simulink subsystem "FTC_UnknownV2"  (R2022a)
settings: Solver=VariableStepAuto  StartTime=0.0  StopTime=10.0  RelTol=1e-3
values from neighbouring files (symbols this model uses):
  g = (9.8)    (= 9.8)    [H250_LOEKnown_400HzParam.m]    (also in H250_LOEUnknown_400HzParam.m; H333_LOEKnown_400HzParam.m)
  J = (diag([0.0056 0.0056 0.0104]))    [H250_LOEKnown_400HzParam.m]    (also in H250_LOEUnknown_400HzParam.m; H333_LOEKnown_400HzParam.m = (diag([0.012 0.0120 0.02])))
  M = ([ 1          1          1         1 ... (first row only)    [H250_LOEKnown_400HzParam.m]    (also in H250_LOEUnknown_400HzParam.m; H333_LOEKnown_400HzParam.m)
  m = (0.752)    (= 0.752)    [H250_LOEKnown_400HzParam.m]    (also in H250_LOEUnknown_400HzParam.m; H333_LOEKnown_400HzParam.m = 1.13)
  MY_ATT_P = Pixhawk_CSC.Parameter( {single(8), 'MY_ATT_P'}  )    [H250_LOEKnown_400HzParam.m]    (also in H250_LOEUnknown_400HzParam.m = Pixhawk_CSC.Parameter( {single(3), 'MY_ATT_P'}  ); H333_LOEKnown_400HzParam.m)
  MY_ATT_P_YAW = Pixhawk_CSC.Parameter( {single(0), 'MY_ATT_P_YAW'}  )    [H250_LOEKnown_400HzParam.m]    (also in H250_LOEUnknown_400HzParam.m = Pixhawk_CSC.Parameter( {single(0.0), 'MY_ATT_P_YAW'}  ); H333_LOEKnown_400HzParam.m)
  MY_K_CP = Pixhawk_CSC.Parameter({single(0.7), 'MY_K_CP'} )    [H250_LOEUnknown_400HzParam.m]
  MY_POS_P = Pixhawk_CSC.Parameter( {single(0.5), 'MY_POS_P'}  )    [H250_LOEKnown_400HzParam.m]    (also in H250_LOEUnknown_400HzParam.m; H333_LOEKnown_400HzParam.m)
  MY_RATE_P = Pixhawk_CSC.Parameter( {single(12), 'MY_RATE_P'}  )    [H250_LOEKnown_400HzParam.m]    (also in H250_LOEUnknown_400HzParam.m = Pixhawk_CSC.Parameter( {single(14), 'MY_RATE_P'}  ); H333_LOEKnown_400HzParam.m)
  MY_RATE_P_YAW = Pixhawk_CSC.Parameter( {single(0.3), 'MY_RATE_P_YAW'}  )    [H250_LOEKnown_400HzParam.m]    (also in H250_LOEUnknown_400HzParam.m = Pixhawk_CSC.Parameter( {single(0.0), 'MY_RATE_P_YAW'}  ); H333_LOEKnown_400HzParam.m)
  MY_SAT_AD = Pixhawk_CSC.Parameter({single(0.13), 'MY_SAT_AD'} )    [H250_LOEKnown_400HzParam.m]    (also in H250_LOEUnknown_400HzParam.m; H333_LOEKnown_400HzParam.m)
  MY_TAU_P_A = Pixhawk_CSC.Parameter( {single(0), 'MY_TAU_P_A'}  )    [H250_LOEKnown_400HzParam.m]    (also in H250_LOEUnknown_400HzParam.m = Pixhawk_CSC.Parameter( {single(0.0), 'MY_TAU_P_A'}  ); H333_LOEKnown_400HzParam.m)
  MY_TAU_P_A_YAW = Pixhawk_CSC.Parameter( {single(0), 'MY_TAU_P_A_YAW'}  )    [H250_LOEKnown_400HzParam.m]    (also in H250_LOEUnknown_400HzParam.m; H333_LOEKnown_400HzParam.m)
  MY_TAU_P_P = Pixhawk_CSC.Parameter( {single(1.5), 'MY_TAU_P_P'}  )    [H250_LOEKnown_400HzParam.m]    (also in H250_LOEUnknown_400HzParam.m = Pixhawk_CSC.Parameter( {single(1.3), 'MY_TAU_P_P'}  ); H333_LOEKnown_400HzParam.m)
  MY_TAU_P_P_YAW = Pixhawk_CSC.Parameter( {single(0.1), 'MY_TAU_P_P_YAW'}  )    [H250_LOEKnown_400HzParam.m]    (also in H250_LOEUnknown_400HzParam.m; H333_LOEKnown_400HzParam.m)
  MY_VEL_P = Pixhawk_CSC.Parameter( {single(0.8), 'MY_VEL_P'}  )    [H250_LOEKnown_400HzParam.m]    (also in H250_LOEUnknown_400HzParam.m; H333_LOEKnown_400HzParam.m)
  T00 = single([m*g/4 m*g/4 m*g/4 m*g/4]')    [H250_LOEKnown_400HzParam.m]    (also in H250_LOEUnknown_400HzParam.m; H333_LOEKnown_400HzParam.m)
  Tf = 0.06    [H250_LOEKnown_400HzParam.m]    (also in H250_LOEUnknown_400HzParam.m; H333_LOEKnown_400HzParam.m)
  Tmotorbar = (0.035)    (= 0.035)    [H250_LOEKnown_400HzParam.m]    (also in H250_LOEUnknown_400HzParam.m = 0.032; H333_LOEKnown_400HzParam.m)
  Ts = 1/400    (= 0.0025)    [H250_LOEKnown_400HzParam.m]    (also in H250_LOEUnknown_400HzParam.m; H333_LOEKnown_400HzParam.m)
undefined symbols (not defined in the file or in its folder): MY_POS_ALT, MY_VEL_ALT
libraries: discretizing x14, slpidlib x4, simulink x2, pixhawk_slib_uORB_RW x1
settings Model: Creator=kcx06  LastModifiedBy=kcx06
settings SolverCC: AlgebraicLoopSolver=TrustRegion
settings DebuggingCC: UnconnectedInputMsg=warning  UnconnectedOutputMsg=warning  UnconnectedLineMsg=warning  SFMachineParentedDataDiag=warning
settings RTWCC: DLArmComputeVersion=19.05

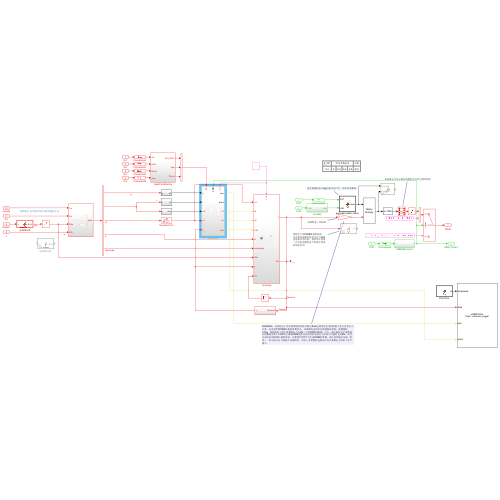
[thumbnail: Simulink's stored preview of the top-level diagram]
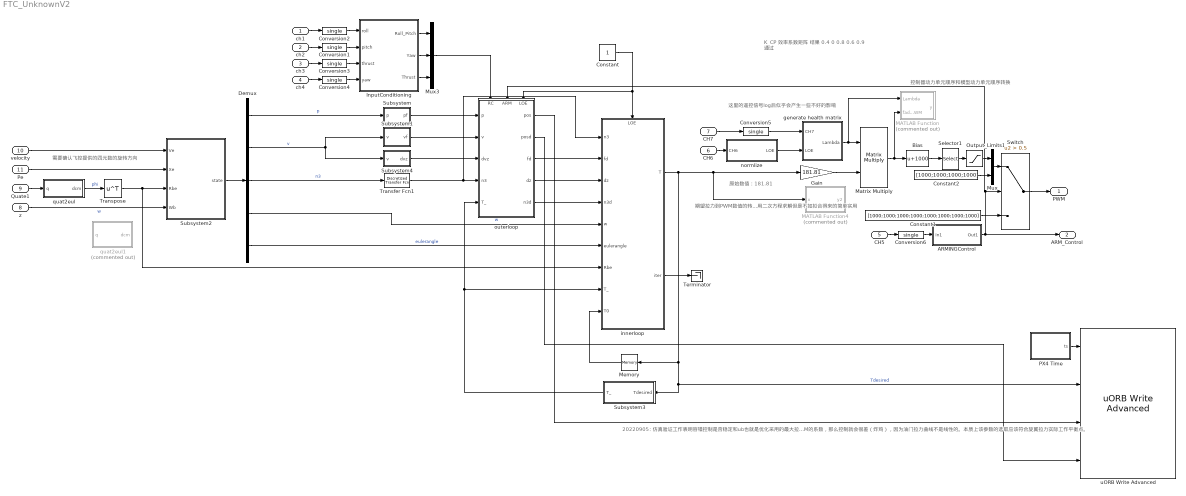
== system FTC_UnknownV2 ==
  note: 这里的遥控信号log后似乎会产生一些不好的影响
  note: K_CP
      | 效率系数矩阵
      | 结果
      |
      | 0.4
      | 0
      | 0.8
      | 0.6
      | 0.9
      | 通过
  note: 20220905：仿真验证工作表明容错控制是否稳定和ub也就是优化采用的最大拉力没有太大关系。而是和T到PWM转换的系数有关，该系数的选取更可能遵循该原则：旋翼整机0.7kg，故障情况下每个旋翼的拉力为2N（大约PWM=1400）左右，那么乘以这个系数的后的数值再加上1000所生成的PWM值所对应的实际电机拉力应该尽可能的也是2N。所以在实际采用8.5N上限的时候，如果使用117作为生成PWM的系数，那么控制就会很差（炸鸡），因为油门拉力曲线不是线性的。本质上该参数的选取应该符合旋翼拉力实际工作平衡点。
  note: 期望拉力到PWM数值的转换，该关系是根据电机油门拉力数据直接拟合得出的。虽然可以使用二次方程求解但是不如拟合得来的简单实用
  note: 原始数值：181.81
  note: 需要确认飞控提供的四元数的旋转方向
  note: 控制器动力单元顺序和模型动力单元顺序转换
  ch1 : Inport  OutDataTypeStr=uint16  PortDimensions=1
  ch2 : Inport  Port=2  OutDataTypeStr=uint16  PortDimensions=1
  ch3 : Inport  Port=3  OutDataTypeStr=uint16  PortDimensions=1
  ch4 : Inport  Port=4  OutDataTypeStr=uint16  PortDimensions=1
  CH5 : Inport  Port=5  OutDataTypeStr=uint16  PortDimensions=1  Interpolate=off
  CH6 : Inport  Port=6
  CH7 : Inport  Port=7
  z : Inport  Port=8
  Quate1 : Inport  Port=9
  velocity : Inport  Port=10
  Pe : Inport  Port=11
  ARMINGControl : Subsystem
  Bias : Bias  Bias=1000  SaturateOnIntegerOverflow=off
  Constant : Constant  OutDataTypeStr=single
  Constant1 : Constant  Value=[1000;1000;1000;1000;1000;1000;1000;1000]  OutDataTypeStr=single
  Constant2 : Constant  Value=[1000;1000;1000;1000]  OutDataTypeStr=single
  Conversion{1..6} (6 alike) : DataTypeConversion  OutDataTypeStr=single  SaturateOnIntegerOverflow=off  RndMeth=Floor
  Demux : Demux  Outputs=[3 3 3 3 3]
  Gain : Gain  Gain=181.81  OutDataTypeStr=single
  InputConditioning : Subsystem
  MATLAB Function : MATLAB Function  Commented=on  TreatAsAtomicUnit=on
  MATLAB Function4 : MATLAB Function  Commented=on  TreatAsAtomicUnit=on
  Matrix Multiply : Product  Multiplication=Matrix(*)
  Memory : Memory  InitialCondition=T00
  Mux : Mux  Inputs=2
  Mux3 : Mux  Inputs=3
  Output_Limits1 : Saturate  UpperLimit=2000  LowerLimit=1000
  PX4 Time : MATLAB Function  TreatAsAtomicUnit=on
  Selector1 : Selector  IndexMode=Zero-based  InputPortWidth=4  IndexOptions=Index vector (dialog)  Indices=[0 2 3 1]  OutputSizes=1
  Subsystem : Subsystem
  Subsystem1 : Subsystem
  Subsystem2 : Subsystem
  Subsystem3 : Subsystem
  Subsystem4 : Subsystem
  Switch : Switch  Criteria=u2 > Threshold  Threshold=0.5  SaturateOnIntegerOverflow=off  InputSameDT=off
  Terminator : Terminator
  Transfer Fcn1 : discretizing/Discretized Transfer Fcn  Numerator=[1]  Denominator=[Tf 1]  AbsTol=auto  SampleTime=Ts  method=zoh  Wc=1
      link override Discrete Transfer Fcn: InitialStates=[0;0;1]
      settings: SourceProductBaseCode=SL
  Transpose : Math  Operator=transpose
  generate health matrix : MATLAB Function  TreatAsAtomicUnit=on
  innerloop : Subsystem
      settings: PortSchema="{\"entries\":[{\"content\":{\"sides\":[{\"content\":{\"connectorIds\":[\"In1\",\"In2\",\"In3\",\"In4\",\"In5\",\"In6\",\"In7\",\"In8\",\"In9\"]},\"type\":\"ConnectorPlacement.EquallySpacedRectSide\",\"uuid\":\"43c6e1bd-c98b-47b4-98da-f51fdffff433\"},{\"content\":{\"connectorIds\":[\"Out1\",\"Out2\"],\"side\":\"RIGHT\"},\"type\":\"ConnectorPlacement.EquallySpacedRectSide\",\"uuid\":\"ac1c9532-9168-4bf4-8fed-08d3fdc16453\"},{\"content\":{\"connectorIds\":[\"In10\"],\"side\":\"TOP\"},\"type\":\"ConnectorPlacement.EquallySpacedRectSide\",\"uuid\":\"32774b13-030c-47c6-b846-fc6c0ce2dd6f\"}]},\"type\":\"ConnectorPlacement.EquallySpacedConnector\",\"uuid\":\"dd62421a-d766-429a-a161-5a0f77c5a7ba\"}],\"packageUris\":[\"http://schema.mathworks.com/mf0/Connector/R2020b\"],\"version\":\"1.0\"}"
  normlize : Subsystem
  outerloop : Subsystem
      settings: PortSchema="{\"entries\":[{\"content\":{\"sides\":[{\"content\":{\"connectorIds\":[\"In1\",\"In2\",\"In3\",\"In4\",\"In5\"]},\"type\":\"ConnectorPlacement.EquallySpacedRectSide\",\"uuid\":\"59983f3e-2daf-41bd-bc3f-074c85f4b2eb\"},{\"content\":{\"connectorIds\":[\"Out1\",\"Out2\",\"Out3\",\"Out4\",\"Out5\"],\"side\":\"RIGHT\"},\"type\":\"ConnectorPlacement.EquallySpacedRectSide\",\"uuid\":\"6ee11e40-7870-4737-b9e6-fd7c25119100\"},{\"content\":{\"connectorIds\":[\"In6\",\"In7\",\"In8\"],\"side\":\"TOP\"},\"type\":\"ConnectorPlacement.EquallySpacedRectSide\",\"uuid\":\"847e9a02-4621-4cf8-a675-1479afa28be0\"}]},\"type\":\"ConnectorPlacement.EquallySpacedConnector\",\"uuid\":\"28981c41-e87e-4da3-ac2d-04a56d75ff2b\"}],\"packageUris\":[\"http://schema.mathworks.com/mf0/Connector/R2020b\"],\"version\":\"1.0\"}"
  quat2eul : MATLAB Function  TreatAsAtomicUnit=on
  quat2eul1 : MATLAB Function  Commented=on  TreatAsAtomicUnit=on
  uORB Write Advanced : pixhawk_slib_uORB_RW/uORB Write Advanced  Ts=0  uORB_AdvtQueue=on  uORB_FieldEnabledArr="0  0  0  1  0  0  0  0  0  0  0"  uORB_Topic_str=0  uORB_Struct_DT="[1  1  1  1  1]"  BlockInputCount=5  uORB_StructParams="[\"voltage_v\",\"voltage_filtered_v\",\"current_a\",\"current_filtered_a\",\"remaining\"]"  uORB_PortSizes="[1  1  1  1]"  MsgSizeOf=0  MW_update=true
      settings: SourceProductName=Pixhawk Target Blocks
  PWM : Outport  PortDimensions=8  VectorParamsAs1DForOutWhenUnconnected=off
  ARM_Control : Outport  Port=2  PortDimensions=1  VectorParamsAs1DForOutWhenUnconnected=off
  wires:
  CH6/1 -> normlize/1(CH6)
  InputConditioning/3(Thrust) -> Mux3/3
  velocity/1 -> Subsystem2/1(Ve)
  Conversion2/1 -> InputConditioning/1(roll)
  Transpose/1 -> innerloop/7(Rbe), Subsystem2/3(Rbe)
  Demux/3 -> Transfer Fcn1/1  "n3"
  InputConditioning/1(Roll_Pitch) -> Mux3/1
  outerloop/4(dz) -> innerloop/3(dz)
  Constant/1 -> outerloop/8(LOE), innerloop/10(LOE)
  Constant1/1 -> Switch/3
  Subsystem3/1(T_) -> outerloop/5(T_), innerloop/8(T_)
  quat2eul/1(dcm) -> Transpose/1  "phi"
  z/1 -> Subsystem2/4(Wb)  "w"
  Conversion3/1 -> InputConditioning/3(thrust)
  Pe/1 -> Subsystem2/2(Xe)
  CH5/1 -> Conversion6/1
  Quate1/1 -> quat2eul/1(q)
  Demux/2 -> Subsystem1/1(v), Subsystem4/1(v)  "v"
  ch4/1 -> Conversion4/1
  Output_Limits1/1 -> Mux/1
  Demux/4 -> innerloop/5(w)  "w"
  outerloop/3(fd) -> innerloop/2(fd)
  Memory/1 -> innerloop/9(T0)
  Demux/5 -> innerloop/6(eulerangle)  "eulerangle"
  ch1/1 -> Conversion2/1
  InputConditioning/2(Yaw) -> Mux3/2
  Selector1/1 -> Output_Limits1/1
  innerloop/1(T) -> Subsystem3/1(Tdesired), uORB Write Advanced/2, Memory/1, Gain/1, MATLAB Function4/1(x)  "Tdesired"
  ch2/1 -> Conversion1/1
  Conversion4/1 -> InputConditioning/4(yaw)
  normlize/1(LOE) -> generate health matrix/2(LOE)
  Mux/1 -> Switch/1
  Subsystem2/1(state) -> Demux/1
  Conversion6/1 -> ARMINGControl/1(In1)
  Switch/1 -> PWM/1
  ch3/1 -> Conversion3/1
  ARMINGControl/1(Out1) -> outerloop/7(ARM), Switch/2, ARM_Control/1
  Mux3/1 -> outerloop/6(RC)
  Constant2/1 -> Mux/2
  Conversion1/1 -> InputConditioning/2(pitch)
  outerloop/5(n3d) -> innerloop/4(n3d)
  Demux/1 -> Subsystem/1(p)  "p"
  Subsystem/1(pf) -> outerloop/1(p)
  Subsystem1/1(vf) -> outerloop/2(v)
  Subsystem4/1(dvz) -> outerloop/3(dvz)
  Transfer Fcn1/1 -> innerloop/1(n3), outerloop/4(n3)
  PX4 Time/1(ts) -> uORB Write Advanced/1
  innerloop/2(iter) -> Terminator/1
  outerloop/1(pos) -> uORB Write Advanced/3
  outerloop/2(posd) -> uORB Write Advanced/4
  Matrix Multiply/1 -> MATLAB Function/2(fadePWM), Bias/1
  Gain/1 -> Matrix Multiply/2
  generate health matrix/1(Lambda) -> MATLAB Function/1(Lambda), Matrix Multiply/1
  CH7/1 -> Conversion5/1
  Conversion5/1 -> generate health matrix/1(CH7)
  Bias/1 -> Selector1/1

== system FTC_UnknownV2/ARMINGControl ==
  In1 : Inport
  Compare To Constant3 : simulink/Logic and Bit Operations/Compare To Constant  relop=>=  const=uint16(1500)  OutDataTypeStr=boolean
  Out1 : Outport  VectorParamsAs1DForOutWhenUnconnected=off
  wires:
  In1/1 -> Compare To Constant3/1
  Compare To Constant3/1 -> Out1/1

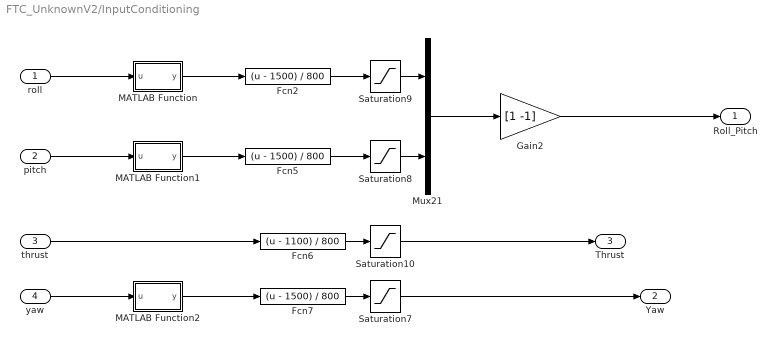
== system FTC_UnknownV2/InputConditioning ==
  roll : Inport
  pitch : Inport  Port=2
  thrust : Inport  Port=3
  yaw : Inport  Port=4
  Fcn2 : Fcn  Expr=(u - 1500) / 800
  Fcn5 : Fcn  Expr=(u - 1500) / 800
  Fcn6 : Fcn  Expr=(u - 1100) / 800
  Fcn7 : Fcn  Expr=(u - 1500) / 800
  Gain2 : Gain  Gain=[1 -1]  OutDataTypeStr=Inherit: Inherit via back propagation
  MATLAB Function : MATLAB Function  TreatAsAtomicUnit=on
  MATLAB Function1 : MATLAB Function  TreatAsAtomicUnit=on
  MATLAB Function2 : MATLAB Function  TreatAsAtomicUnit=on
  Mux21 : Mux  Inputs=2
  Saturation10 : Saturate  UpperLimit=1  LowerLimit=0
  Saturation7 : Saturate  UpperLimit=1  LowerLimit=-1
  Saturation8 : Saturate  UpperLimit=1  LowerLimit=-1
  Saturation9 : Saturate  UpperLimit=1  LowerLimit=-1
  Roll_Pitch : Outport  VectorParamsAs1DForOutWhenUnconnected=off
  Yaw : Outport  Port=2  VectorParamsAs1DForOutWhenUnconnected=off
  Thrust : Outport  Port=3  VectorParamsAs1DForOutWhenUnconnected=off
  wires:
  yaw/1 -> MATLAB Function2/1(u)
  MATLAB Function/1(y) -> Fcn2/1
  MATLAB Function1/1(y) -> Fcn5/1
  roll/1 -> MATLAB Function/1(u)
  thrust/1 -> Fcn6/1
  MATLAB Function2/1(y) -> Fcn7/1
  pitch/1 -> MATLAB Function1/1(u)
  Fcn7/1 -> Saturation7/1
  Saturation9/1 -> Mux21/1
  Fcn5/1 -> Saturation8/1
  Fcn2/1 -> Saturation9/1
  Fcn6/1 -> Saturation10/1
  Saturation8/1 -> Mux21/2
  Mux21/1 -> Gain2/1
  Gain2/1 -> Roll_Pitch/1
  Saturation7/1 -> Yaw/1
  Saturation10/1 -> Thrust/1

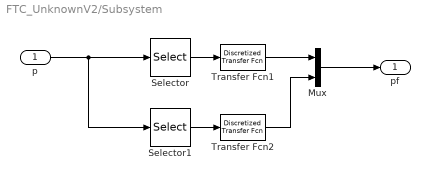
== system FTC_UnknownV2/Subsystem ==
  p : Inport
  Mux : Mux  Inputs=2
  Selector : Selector  IndexMode=Zero-based  InputPortWidth=3  IndexOptions=Index vector (dialog)  Indices=[0 1]  OutputSizes=1
  Selector1 : Selector  IndexMode=Zero-based  InputPortWidth=3  IndexOptions=Index vector (dialog)  Indices=[2]  OutputSizes=1
  Transfer Fcn1 : discretizing/Discretized Transfer Fcn  Numerator=[1 ]  Denominator=[Tf 1]  AbsTol=auto  SampleTime=Ts  method=zoh  Wc=1
      settings: SourceProductBaseCode=SL
  Transfer Fcn2 : discretizing/Discretized Transfer Fcn  Numerator=[1 ]  Denominator=[Tf 1]  AbsTol=auto  SampleTime=Ts  method=zoh  Wc=1
      settings: SourceProductBaseCode=SL
  pf : Outport
  wires:
  Transfer Fcn1/1 -> Mux/1
  Selector/1 -> Transfer Fcn1/1
  Transfer Fcn2/1 -> Mux/2
  Selector1/1 -> Transfer Fcn2/1
  Mux/1 -> pf/1
  p/1 -> Selector/1, Selector1/1

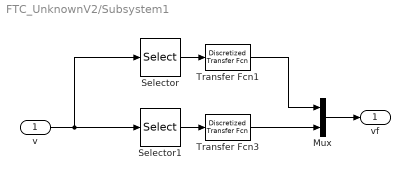
== system FTC_UnknownV2/Subsystem1 ==
  v : Inport
  Mux : Mux  Inputs=2
  Selector : Selector  IndexMode=Zero-based  InputPortWidth=3  IndexOptions=Index vector (dialog)  Indices=[0 1]  OutputSizes=1
  Selector1 : Selector  IndexMode=Zero-based  InputPortWidth=3  IndexOptions=Index vector (dialog)  Indices=[2]  OutputSizes=1
  Transfer Fcn1 : discretizing/Discretized Transfer Fcn  Numerator=[1 ]  Denominator=[Tf 1]  AbsTol=auto  SampleTime=Ts  method=zoh  Wc=1
      settings: SourceProductBaseCode=SL
  Transfer Fcn3 : discretizing/Discretized Transfer Fcn  Numerator=[1 ]  Denominator=[Tf 1]  AbsTol=auto  SampleTime=Ts  method=zoh  Wc=1
      settings: SourceProductBaseCode=SL
  vf : Outport
  wires:
  Transfer Fcn1/1 -> Mux/1
  Selector/1 -> Transfer Fcn1/1
  Mux/1 -> vf/1
  v/1 -> Selector1/1, Selector/1
  Selector1/1 -> Transfer Fcn3/1
  Transfer Fcn3/1 -> Mux/2

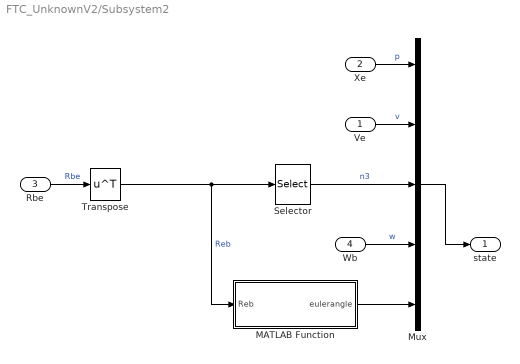
== system FTC_UnknownV2/Subsystem2 ==
  Ve : Inport
  Xe : Inport  Port=2
  Rbe : Inport  Port=3
  Wb : Inport  Port=4
  MATLAB Function : MATLAB Function  TreatAsAtomicUnit=on
  Mux : Mux  Inputs=[3 3 3 3 3]
  Selector : Selector  NumberOfDimensions=2  IndexMode=Zero-based  InputPortWidth=3  IndexOptions=Select all,Index vector (dialog)  Indices=[1 3],2  OutputSizes=1,1
  Transpose : Math  Operator=transpose
  state : Outport
  wires:
  Transpose/1 -> MATLAB Function/1(Reb), Selector/1  "Reb"
  Xe/1 -> Mux/1  "p"
  Ve/1 -> Mux/2  "v"
  Wb/1 -> Mux/4  "w"
  Selector/1 -> Mux/3  "n3"
  Rbe/1 -> Transpose/1  "Rbe"
  MATLAB Function/1(eulerangle) -> Mux/5
  Mux/1 -> state/1

== system FTC_UnknownV2/Subsystem3 ==
  Tdesired : Inport
  Transfer Fcn10 : discretizing/Discretized Transfer Fcn  Numerator=[1]  Denominator=[Tmotorbar 1]  AbsTol=auto  SampleTime=Ts  method=zoh  Wc=1
      settings: SourceProductBaseCode=SL
  Transfer Fcn9 : discretizing/Discretized Transfer Fcn  Numerator=[1]  Denominator=[Tf 1]  AbsTol=auto  SampleTime=Ts  method=zoh  Wc=1
      settings: SourceProductBaseCode=SL
  T_ : Outport
  wires:
  Transfer Fcn9/1 -> Transfer Fcn10/1
  Tdesired/1 -> Transfer Fcn9/1
  Transfer Fcn10/1 -> T_/1

== system FTC_UnknownV2/Subsystem4 ==
  v : Inport
  Selector2 : Selector  IndexMode=Zero-based  InputPortWidth=3  IndexOptions=Index vector (dialog)  Indices=[2]  OutputSizes=1
  Transfer Fcn : discretizing/Discretized Transfer Fcn  Numerator=[1 0]  Denominator=[Tf 1]  AbsTol=auto  SampleTime=Ts  method=zoh  Wc=1
      settings: SourceProductBaseCode=SL
  dvz : Outport
  wires:
  Transfer Fcn/1 -> dvz/1
  v/1 -> Selector2/1
  Selector2/1 -> Transfer Fcn/1

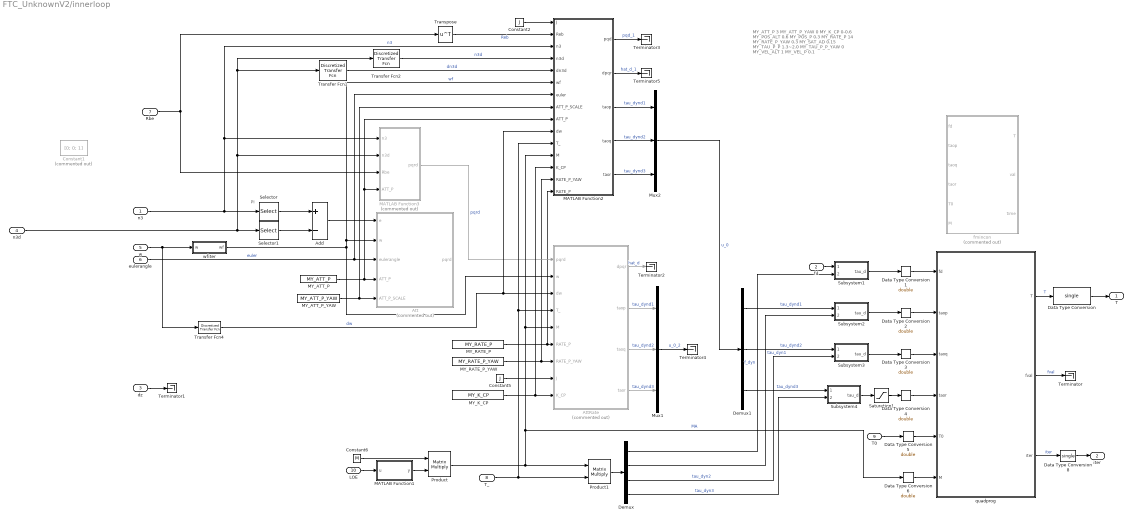
== system FTC_UnknownV2/innerloop ==
  note: PI
  note: MY_ATT_P
      | 3
      |
      | MY_ATT_P_YAW
      | 0
      |
      | MY_K_CP
      | 0-0.6
      |
      | MY_POS_ALT
      | 0.6
      |
      | MY_POS_P
      | 0.3
      |
      | MY_RATE_P
      | 14
      |
      | MY_RATE_P_YAW
      | 0.3
      |
      | MY_SAT_AD
      | 0.15
      |
      | MY_TAU_P_P
      | 1.3~2.0
      |
      | MY_TAU_P_P_YAW
      | 0
      |
      | MY_VEL_ALT
      | 1
      |
      | MY_VEL_P
      | 0.1
  n3 : Inport
  fd : Inport  Port=2
  dz : Inport  Port=3
  n3d : Inport  Port=4
  w : Inport  Port=5
  eulerangle : Inport  Port=6
  Rbe : Inport  Port=7
  T_ : Inport  Port=8
  T0 : Inport  Port=9
  LOE : Inport  Port=10
  Add : Sum  Inputs=+-
  Att : MATLAB Function  Commented=on  TreatAsAtomicUnit=on
  AttRate : MATLAB Function  Commented=on  TreatAsAtomicUnit=on
  Constant1 : Constant  Commented=on  Value=[0; 0; 1]
  Constant2 : Constant  Value=J  OutDataTypeStr=single
  Constant5 : Constant  Value=J  OutDataTypeStr=single
  Constant6 : Constant  Value=M  OutDataTypeStr=single
  Data Type Conversion : DataTypeConversion  OutDataTypeStr=single  SaturateOnIntegerOverflow=off  RndMeth=Floor
  Data Type Conversion{1..6} (6 alike) : DataTypeConversion  OutDataTypeStr=double  SaturateOnIntegerOverflow=off  RndMeth=Floor
  Data Type Conversion8 : DataTypeConversion  OutDataTypeStr=single  SaturateOnIntegerOverflow=off  RndMeth=Floor
  Demux : Demux
  Demux1 : Demux  Outputs=3
  MATLAB Function1 : MATLAB Function  TreatAsAtomicUnit=on
  MATLAB Function2 : MATLAB Function  TreatAsAtomicUnit=on
  MATLAB Function3 : MATLAB Function  Commented=on  TreatAsAtomicUnit=on
  MY_ATT_P : Constant  Value=MY_ATT_P
  MY_ATT_P_YAW : Constant  Value=MY_ATT_P_YAW
  MY_K_CP : Constant  Value=MY_K_CP
  MY_RATE_P : Constant  Value=MY_RATE_P
  MY_RATE_P_YAW : Constant  Value=MY_RATE_P_YAW
  Mux1 : Mux  Inputs=3
  Mux2 : Mux  Inputs=3
  Product : Product  Multiplication=Matrix(*)
  Product1 : Product  Multiplication=Matrix(*)
  Saturation1 : Saturate  UpperLimit=0.075  LowerLimit=-0.075
  Selector : Selector  IndexMode=Zero-based  InputPortWidth=3  IndexOptions=Index vector (dialog)  Indices=[0 1]  OutputSizes=1
  Selector1 : Selector  IndexMode=Zero-based  InputPortWidth=3  IndexOptions=Index vector (dialog)  Indices=[0 1]  OutputSizes=1
  Subsystem1 : Subsystem
  Subsystem2 : Subsystem
  Subsystem3 : Subsystem
  Subsystem4 : Subsystem
  Terminator{,1..5} (6 alike) : Terminator
  Transfer Fcn1 : discretizing/Discretized Transfer Fcn  Numerator=[1 0]  Denominator=[Tf 1]  AbsTol=auto  SampleTime=Ts  method=zoh  Wc=1
      settings: SourceProductBaseCode=SL
  Transfer Fcn2 : discretizing/Discretized Transfer Fcn  Numerator=[1]  Denominator=[Tf 1]  AbsTol=auto  SampleTime=Ts  method=zoh  Wc=1
      link override Discrete Transfer Fcn: InitialStates=[0;0;1]
      settings: SourceProductBaseCode=SL
  Transfer Fcn4 : discretizing/Discretized Transfer Fcn  Numerator=[1 0]  Denominator=[Tf 1]  AbsTol=auto  SampleTime=Ts  method=zoh  Wc=1
      settings: SourceProductBaseCode=SL
  Transpose : Math  Operator=transpose
  fmincon : MATLAB Function  Commented=on  TreatAsAtomicUnit=on
  quadprog : MATLAB Function  TreatAsAtomicUnit=on
  wfiter : Subsystem
  T : Outport  PortDimensions=4
  iter : Outport  Port=2
  wires:
  Mux1/1 -> Terminator4/1  "u_0_2"
  MATLAB Function2/1(pqd) -> Terminator3/1  "pqd_1"
  AttRate/1(dpqr) -> Terminator2/1  "hat_d"
  Mux2/1 -> Demux1/1  "u_0"
  MATLAB Function2/5(taor) -> Mux2/3  "tau_dynd3"
  MATLAB Function2/4(taoq) -> Mux2/2  "tau_dynd2"
  MATLAB Function2/3(taop) -> Mux2/1  "tau_dynd1"
  AttRate/2(taop) -> Mux1/1  "tau_dynd1"
  AttRate/3(taoq) -> Mux1/2  "tau_dynd2"
  AttRate/4(taor) -> Mux1/3  "tau_dynd3"
  Constant2/1 -> MATLAB Function2/1(J)
  Transpose/1 -> MATLAB Function2/2(Reb)  "Reb"
  dz/1 -> Terminator1/1
  Selector/1 -> Add/1
  Selector1/1 -> Add/2
  Rbe/1 -> MATLAB Function3/3(Rbe), Transpose/1
  n3d/1 -> Selector1/1, MATLAB Function3/2(n3d), Transfer Fcn2/1, Transfer Fcn1/1
  MY_ATT_P_YAW/1 -> Att/5(ATT_P_SCALE), MATLAB Function2/8(ATT_P_SCALE)
  MY_ATT_P/1 -> Att/4(ATT_P), MATLAB Function2/9(ATT_P), MATLAB Function3/4(ATT_P)
  MY_RATE_P_YAW/1 -> AttRate/7(RATE_P_YAW), MATLAB Function2/14(RATE_P_YAW)
  MY_RATE_P/1 -> AttRate/6(RATE_P), MATLAB Function2/15(RATE_P)
  Data Type Conversion/1 -> T/1
  MATLAB Function1/1(y) -> Product/2
  MATLAB Function3/1(pqrd) -> AttRate/1(pqrd)  "pqrd"
  Product1/1 -> Demux/1
  n3/1 -> MATLAB Function2/3(n3), MATLAB Function3/1(n3), Selector/1  "n3"
  Product/1 -> Product1/1, AttRate/5(M), MATLAB Function2/12(M), Data Type Conversion6/1  "MA"
  LOE/1 -> MATLAB Function1/1(u)
  Demux/4 -> Subsystem4/2(tau_dyn)  "tau_dyn3"
  Demux1/3 -> Subsystem4/1(tau_dynd)  "tau_dynd3"
  Demux/3 -> Subsystem3/2(tau_dyn)  "tau_dyn2"
  Demux1/2 -> Subsystem3/1(tau_dynd)  "tau_dynd2"
  Demux/2 -> Subsystem2/2(tau_dyn)  "tau_dyn1"
  Demux1/1 -> Subsystem2/1(tau_dynd)  "tau_dynd1"
  fd/1 -> Subsystem1/1(tau_dynd)
  Demux/1 -> Subsystem1/2(tau_dyn)  "f_dyn"
  Data Type Conversion8/1 -> iter/1
  quadprog/3(iter) -> Data Type Conversion8/1  "iter"
  Subsystem4/1(tau_d) -> Saturation1/1
  Data Type Conversion6/1 -> quadprog/6(M)
  Data Type Conversion5/1 -> quadprog/5(T0)
  Data Type Conversion4/1 -> quadprog/4(taor)
  Data Type Conversion3/1 -> quadprog/3(taoq)
  Data Type Conversion2/1 -> quadprog/2(taop)
  Data Type Conversion1/1 -> quadprog/1(fd)
  quadprog/1(T) -> Data Type Conversion/1  "T"
  wfiter/1(wf) -> AttRate/2(w), Att/2(w), MATLAB Function2/6(wf)  "wf"
  w/1 -> Transfer Fcn4/1, wfiter/1(w)
  eulerangle/1 -> Att/3(eulerangle), MATLAB Function2/7(euler)  "euler"
  quadprog/2(fval) -> Terminator/1  "fval"
  Constant6/1 -> Product/1
  Constant5/1 -> AttRate/8(J)
  T_/1 -> AttRate/4(T_), MATLAB Function2/11(T_), Product1/2
  T0/1 -> Data Type Conversion5/1
  MATLAB Function2/2(dpqr) -> Terminator5/1  "hat_d_1"
  Transfer Fcn4/1 -> AttRate/3(dw), MATLAB Function2/10(dw)  "dw"
  MY_K_CP/1 -> AttRate/9(K_CP), MATLAB Function2/13(K_CP)
  Add/1 -> Att/1(e)
  Subsystem1/1(tau_d) -> Data Type Conversion1/1
  Subsystem2/1(tau_d) -> Data Type Conversion2/1
  Subsystem3/1(tau_d) -> Data Type Conversion3/1
  Saturation1/1 -> Data Type Conversion4/1
  Transfer Fcn2/1 -> MATLAB Function2/4(n3d)  "n3d"
  Transfer Fcn1/1 -> MATLAB Function2/5(dn3d)  "dn3d"

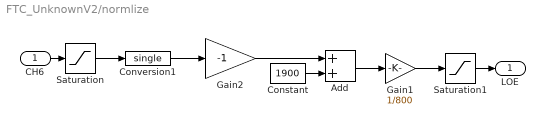
== system FTC_UnknownV2/normlize ==
  CH6 : Inport
  Add : Sum
  Constant : Constant  Value=1900  OutDataTypeStr=single
  Conversion1 : DataTypeConversion  OutDataTypeStr=single  SaturateOnIntegerOverflow=off  RndMeth=Floor
  Gain1 : Gain  Gain=1/800
  Gain2 : Gain  Gain=-1
  Saturation : Saturate  UpperLimit=1900  LowerLimit=1100
  Saturation1 : Saturate  UpperLimit=1  LowerLimit=0
  LOE : Outport
  wires:
  Saturation1/1 -> LOE/1
  Conversion1/1 -> Gain2/1
  Constant/1 -> Add/2
  CH6/1 -> Saturation/1
  Add/1 -> Gain1/1
  Gain1/1 -> Saturation1/1
  Gain2/1 -> Add/1
  Saturation/1 -> Conversion1/1

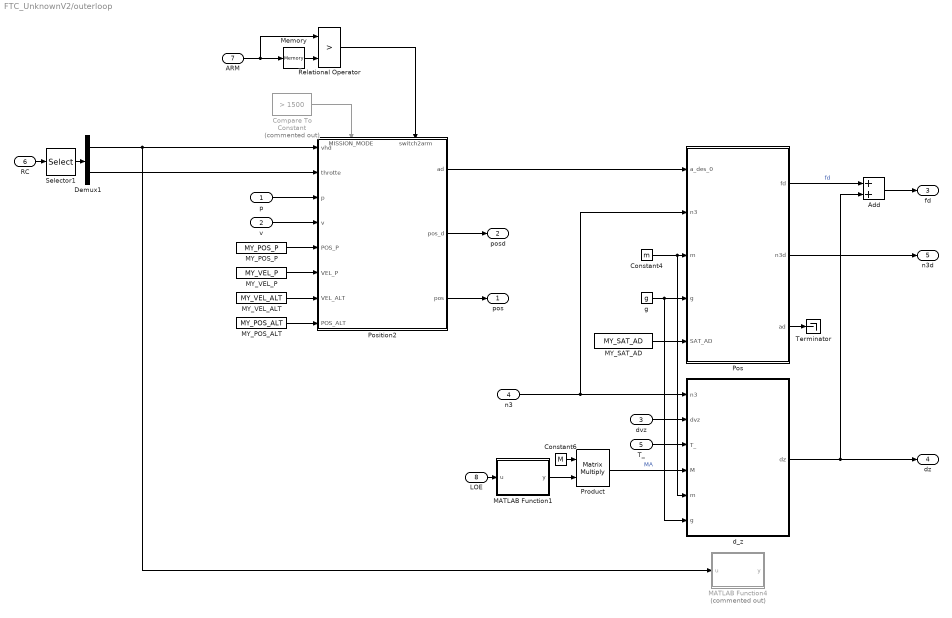
== system FTC_UnknownV2/outerloop ==
  p : Inport
  v : Inport  Port=2
  dvz : Inport  Port=3
  n3 : Inport  Port=4
  T_ : Inport  Port=5
  RC : Inport  Port=6
  ARM : Inport  Port=7
  LOE : Inport  Port=8
  Add : Sum
  Compare To Constant : simulink/Logic and Bit Operations/Compare To Constant  Commented=on  relop=>  const=1500  OutDataTypeStr=boolean
  Constant4 : Constant  Value=m  OutDataTypeStr=single
  Constant6 : Constant  Value=M  OutDataTypeStr=single
  Demux1 : Demux  Outputs=[2 1]
  MATLAB Function1 : MATLAB Function  TreatAsAtomicUnit=on
  MATLAB Function4 : MATLAB Function  Commented=on  TreatAsAtomicUnit=on
  MY_POS_ALT : Constant  Value=MY_POS_ALT
  MY_POS_P : Constant  Value=MY_POS_P
  MY_SAT_AD : Constant  Value=MY_SAT_AD
      settings: AttributesFormatString=|
      | 0.13
      | Default
  MY_VEL_ALT : Constant  Value=MY_VEL_ALT
  MY_VEL_P : Constant  Value=MY_VEL_P
  Memory : Memory  InheritSampleTime=on
  Pos : MATLAB Function  TreatAsAtomicUnit=on
  Position2 : Subsystem
      settings: PortSchema="{\"entries\":[{\"content\":{\"sides\":[{\"content\":{\"connectorIds\":[\"In1\",\"In2\",\"In3\",\"In4\",\"In5\",\"In6\",\"In7\",\"In8\"]},\"type\":\"ConnectorPlacement.EquallySpacedRectSide\",\"uuid\":\"60776ec6-01a0-44f3-b730-3d7732f047d0\"},{\"content\":{\"connectorIds\":[\"Out1\",\"Out2\",\"Out3\"],\"side\":\"RIGHT\"},\"type\":\"ConnectorPlacement.EquallySpacedRectSide\",\"uuid\":\"42b0027c-881e-456b-a4a1-739d1f8a7516\"},{\"content\":{\"connectorIds\":[\"In9\",\"In10\"],\"side\":\"TOP\"},\"type\":\"ConnectorPlacement.EquallySpacedRectSide\",\"uuid\":\"cc212ab2-5a31-41d0-b525-290641d80c94\"}]},\"type\":\"ConnectorPlacement.EquallySpacedConnector\",\"uuid\":\"907853b4-a5dd-49ed-90eb-6ed189df5e2d\"}],\"packageUris\":[\"http://schema.mathworks.com/mf0/Connector/R2020b\"],\"version\":\"1.0\"}"
  Product : Product  Multiplication=Matrix(*)
  Relational Operator : RelationalOperator  Operator=>  OutDataTypeStr=boolean  RndMeth=Simplest  InputSameDT=off
  Selector1 : Selector  IndexMode=Zero-based  InputPortWidth=4  IndexOptions=Index vector (dialog)  Indices=[1 0 3]  OutputSizes=1
  Terminator : Terminator
  d_z : MATLAB Function  TreatAsAtomicUnit=on
  g : Constant  Value=g  OutDataTypeStr=single
  pos : Outport
  posd : Outport  Port=2
  fd : Outport  Port=3
  dz : Outport  Port=4
  n3d : Outport  Port=5
  wires:
  Pos/2(n3d) -> n3d/1
  Relational Operator/1 -> Position2/10(switch2arm)
  Memory/1 -> Relational Operator/2
  ARM/1 -> Memory/1, Relational Operator/1
  Compare To Constant/1 -> Position2/9(MISSION_MODE)
  MY_POS_ALT/1 -> Position2/8(POS_ALT)
  MY_VEL_ALT/1 -> Position2/7(VEL_ALT)
  dvz/1 -> d_z/2(dvz)
  p/1 -> Position2/3(p)
  v/1 -> Position2/4(v)
  MY_SAT_AD/1 -> Pos/5(SAT_AD)
  MY_VEL_P/1 -> Position2/6(VEL_P)
  MY_POS_P/1 -> Position2/5(POS_P)
  Demux1/1 -> MATLAB Function4/1(u), Position2/1(vhd)
  Position2/1(ad) -> Pos/1(a_des_0)
  RC/1 -> Selector1/1
  Product/1 -> d_z/4(M)  "MA"
  Constant6/1 -> Product/1
  LOE/1 -> MATLAB Function1/1(u)
  MATLAB Function1/1(y) -> Product/2
  n3/1 -> d_z/1(n3), Pos/2(n3)
  d_z/1(dz) -> Add/2, dz/1
  Add/1 -> fd/1
  g/1 -> d_z/6(g), Pos/4(g)
  Constant4/1 -> d_z/5(m), Pos/3(m)
  T_/1 -> d_z/3(T_)
  Pos/1(fd) -> Add/1  "fd"
  Position2/2(pos_d) -> posd/1
  Position2/3(pos) -> pos/1
  Pos/3(ad) -> Terminator/1
  Selector1/1 -> Demux1/1
  Demux1/2 -> Position2/2(throtte)

== system FTC_UnknownV2/innerloop/Subsystem1 ==
  tau_dynd : Inport
  tau_dyn : Inport  Port=2
  Gain7 : Gain
  Sum1 : Sum  Inputs=|++
  Sum4 : Sum  Inputs=|+-
  tau_d : Outport
  wires:
  tau_dyn/1 -> Sum4/2, Sum1/2
  Sum1/1 -> tau_d/1
  Sum4/1 -> Gain7/1
  Gain7/1 -> Sum1/1
  tau_dynd/1 -> Sum4/1  "omega"

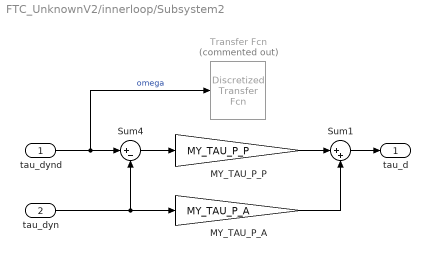
== system FTC_UnknownV2/innerloop/Subsystem2 ==
  tau_dynd : Inport
  tau_dyn : Inport  Port=2
  MY_TAU_P_A : Gain  Gain=MY_TAU_P_A
  MY_TAU_P_P : Gain  Gain=MY_TAU_P_P
  Sum1 : Sum  Inputs=|++
  Sum4 : Sum  Inputs=|+-
  Transfer Fcn : discretizing/Discretized Transfer Fcn  Commented=on  Numerator=[0.005 0]  Denominator=[Tf 1]  AbsTol=auto  SampleTime=Ts  method=zoh  Wc=1
      settings: SourceProductBaseCode=SL
  tau_d : Outport
  wires:
  MY_TAU_P_P/1 -> Sum1/1
  MY_TAU_P_A/1 -> Sum1/2
  tau_dynd/1 -> Sum4/1, Transfer Fcn/1  "omega"
  Sum4/1 -> MY_TAU_P_P/1
  Sum1/1 -> tau_d/1
  tau_dyn/1 -> MY_TAU_P_A/1, Sum4/2

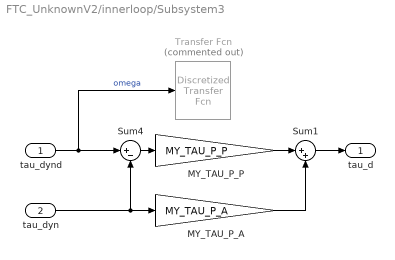
== system FTC_UnknownV2/innerloop/Subsystem3 ==
  tau_dynd : Inport
  tau_dyn : Inport  Port=2
  MY_TAU_P_A : Gain  Gain=MY_TAU_P_A
  MY_TAU_P_P : Gain  Gain=MY_TAU_P_P
  Sum1 : Sum  Inputs=|++
  Sum4 : Sum  Inputs=|+-
  Transfer Fcn : discretizing/Discretized Transfer Fcn  Commented=on  Numerator=[0.005 0]  Denominator=[Tf 1]  AbsTol=auto  SampleTime=Ts  method=zoh  Wc=1
      settings: SourceProductBaseCode=SL
  tau_d : Outport
  wires:
  MY_TAU_P_P/1 -> Sum1/1
  MY_TAU_P_A/1 -> Sum1/2
  tau_dyn/1 -> MY_TAU_P_A/1, Sum4/2
  Sum1/1 -> tau_d/1
  Sum4/1 -> MY_TAU_P_P/1
  tau_dynd/1 -> Sum4/1, Transfer Fcn/1  "omega"

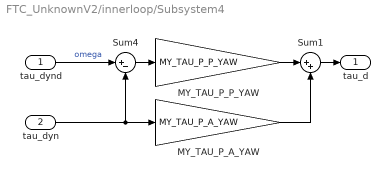
== system FTC_UnknownV2/innerloop/Subsystem4 ==
  tau_dynd : Inport
  tau_dyn : Inport  Port=2
  MY_TAU_P_A_YAW : Gain  Gain=MY_TAU_P_A_YAW
  MY_TAU_P_P_YAW : Gain  Gain=MY_TAU_P_P_YAW
  Sum1 : Sum  Inputs=|++
  Sum4 : Sum  Inputs=|+-
  tau_d : Outport
  wires:
  MY_TAU_P_A_YAW/1 -> Sum1/2
  tau_dynd/1 -> Sum4/1  "omega"
  MY_TAU_P_P_YAW/1 -> Sum1/1
  Sum4/1 -> MY_TAU_P_P_YAW/1
  Sum1/1 -> tau_d/1
  tau_dyn/1 -> Sum4/2, MY_TAU_P_A_YAW/1

== system FTC_UnknownV2/innerloop/wfiter ==
  w : Inport
  Transfer Fcn4 : discretizing/Discretized Transfer Fcn  Numerator=[1]  Denominator=[Tf 1]  AbsTol=auto  SampleTime=Ts  method=zoh  Wc=1
      settings: SourceProductBaseCode=SL
  wf : Outport
  wires:
  w/1 -> Transfer Fcn4/1
  Transfer Fcn4/1 -> wf/1

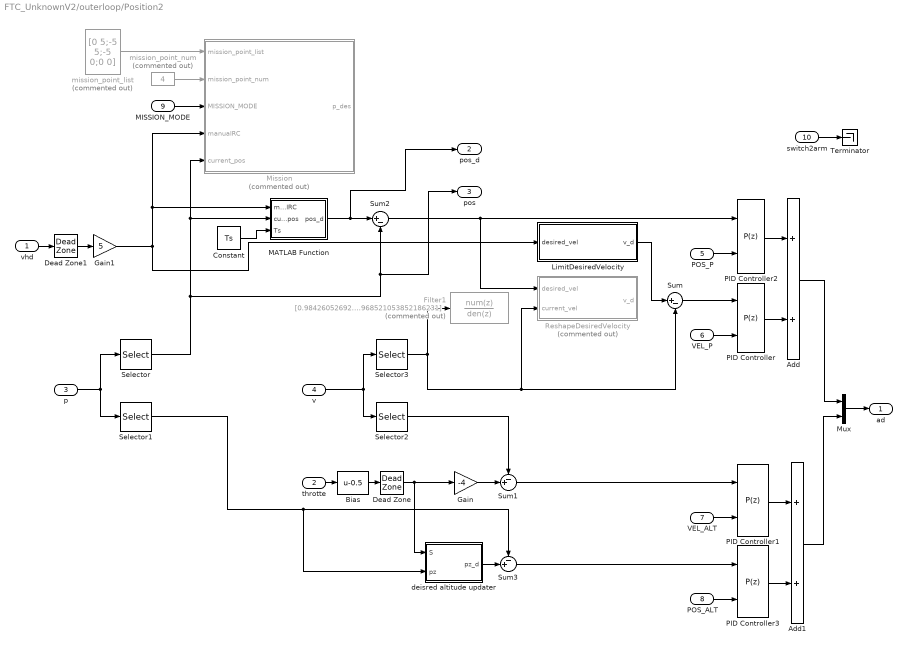
== system FTC_UnknownV2/outerloop/Position2 ==
  vhd : Inport
  throtte : Inport  Port=2
  p : Inport  Port=3
  v : Inport  Port=4
  POS_P : Inport  Port=5
  VEL_P : Inport  Port=6
  VEL_ALT : Inport  Port=7
  POS_ALT : Inport  Port=8
  MISSION_MODE : Inport  Port=9
  switch2arm : Inport  Port=10
  Add : Sum
  Add1 : Sum
  Bias : Bias  Bias=-0.5  SaturateOnIntegerOverflow=off
  Constant : Constant  Value=Ts  OutDataTypeStr=single
  Dead Zone : DeadZone  LowerValue=-0.1  UpperValue=0.1
  Dead Zone1 : DeadZone  LowerValue=-0.1  UpperValue=0.1
  Filter1 : DiscreteFilter  Tag=BlockMethodSubSystem  Commented=on  Numerator=[0.984260526926093116 -1.90667634508841477 0.984260526926093116]  Denominator=[1 -1.90667634508841477 0.968521053852186231]  SampleTime=1/100  a0EqualsOne=on
  Gain : Gain  Gain=-4
  Gain1 : Gain  Gain=5
  LimitDesiredVelocity : MATLAB Function  TreatAsAtomicUnit=on
  MATLAB Function : MATLAB Function  TreatAsAtomicUnit=on
  Mission : Stateflow chart  Commented=on  TreatAsAtomicUnit=on
  Mux : Mux  Inputs=2
  PID Controller{,1..3} (4 alike) : slpidlib/PID Controller  Controller=P  Form=Parallel  TimeDomain=Discrete-time  UseExternalTs=off  SampleTime=-1  IntegratorMethod=Forward Euler  FilterMethod=Forward Euler  ControllerParametersSource=external  P=1  I=1  UseKiTs=on  D=0  N=100  UseFilter=on  TunerSelectOption=Transfer Function Based (PID Tuner App)  InitialConditionSource=internal  InitialConditionForIntegrator=0  InitialConditionForFilter=0  DifferentiatorICPrevScaledInput=0  ExternalReset=none  TrackingMode=off  Kt=1  LimitOutput=off  SatLimitsSource=internal  UpperSaturationLimit=1  LowerSaturationLimit=-1  LinearizeAsGain=on  AntiWindupMode=clamping  Kb=1  POutMin=[]  POutMax=[]  IOutMin=[]  IOutMax=[]  DOutMin=[]  DOutMax=[]  NOutMin=[]  NOutMax=[]  SumOutMin=[]  SumOutMax=[]  SaturationOutMin=[]  SaturationOutMax=[]  PParamMin=[]  PParamMax=[]  IParamMin=[]  IParamMax=[]  DParamMin=[]  DParamMax=[]  NParamMin=[]  NParamMax=[]  KbParamMin=[]  KbParamMax=[]  KtParamMin=[]  KtParamMax=[]  KbOutMin=[]  KbOutMax=[]  KtOutMin=[]  KtOutMax=[]  IntegratorOutMin=[]  IntegratorOutMax=[]  FilterOutMin=[]  FilterOutMax=[]  SumI1OutMin=[]  SumI1OutMax=[]  SumI2OutMin=[]  SumI2OutMax=[]  SumI3OutMin=[]  SumI3OutMax=[]  SumI4OutMin=[]  SumI4OutMax=[]  SumDOutMin=[]  SumDOutMax=[]  DifferentiatorOutMin=[]  DifferentiatorOutMax=[]  FilterDiffOutCoefMin=[]  FilterDiffOutCoefMax=[]  ReciprocalOutMin=[]  ReciprocalOutMax=[]  SumDenOutMin=[]  SumDenOutMax=[]  SumNumOutMin=[]  SumNumOutMax=[]  DivideOutMin=[]  DivideOutMax=[]  UdiffTsProdOutMin=[]  UdiffTsProdOutMax=[]  NTsProdOutMin=[]  NTsProdOutMax=[]  UintegralTsProdOutMin=[]  UintegralTsProdOutMax=[]  UngainTsProdOutMin=[]  UngainTsProdOutMax=[]  IntegratorContinuousStateAttributes=''  IntegratorStateMustResolveToSignalObject=off  IntegratorRTWStateStorageClass=Auto  FilterContinuousStateAttributes=''  FilterStateMustResolveToSignalObject=off  FilterRTWStateStorageClass=Auto  ParallelPVariant=ExternalParameters  IdealPVariant=Disabled  IVariant=Disabled  DVariant=Disabled  IntegratorVariant=Disabled  SatVariant=Disabled  AWVariant=Disabled  PCopyVariant=Disabled  TRVariant=Disabled  FdbkBlocksVariant=Forward  IdealPFdbkVariant=Disabled  SatFdbkVariant=Disabled  DerivativeFilterVariant=Disabled  NVariant=Disabled  NCopyVariant=Disabled_SignalSpec  FilterICVariant=Disabled  IntegratorICVariant=Disabled  ExternalResetVariant=Disabled  TRSumVariant=Passthrough  SumFdbkVariant=Disabled  SumVariant=Passthrough_P  TsampFilterVariant=InternalTs  TsampNgainVariant=Passthrough  TsampIntegralVariant=Disabled_SignalSpec  ExternalSaturationOutDataTypeStr=Inherit: Same as second input  aMode=0
  ReshapeDesiredVelocity : MATLAB Function  Commented=on  TreatAsAtomicUnit=on
  Selector : Selector  InputPortWidth=3  IndexOptions=Index vector (dialog)  Indices=[1 2]  OutputSizes=1
  Selector1 : Selector  InputPortWidth=3  IndexOptions=Index vector (dialog)  Indices=[3]  OutputSizes=1
  Selector2 : Selector  InputPortWidth=3  IndexOptions=Index vector (dialog)  Indices=[3]  OutputSizes=1
  Selector3 : Selector  InputPortWidth=3  IndexOptions=Index vector (dialog)  Indices=[1 2]  OutputSizes=1
  Sum : Sum  Inputs=|+-
  Sum1 : Sum  Inputs=-+|
  Sum2 : Sum  Inputs=|+-
  Sum3 : Sum  Inputs=-+|
  Terminator : Terminator
  deisred altitude updater : MATLAB Function  TreatAsAtomicUnit=on
  mission_point_list : Constant  Commented=on  Value=[0 5;-5 5;-5 0;0 0]  OutDataTypeStr=single
  mission_point_num : Constant  Commented=on  Value=4
  ad : Outport
  pos_d : Outport  Port=2
  pos : Outport  Port=3
  wires:
  Constant/1 -> MATLAB Function/3(Ts)
  MATLAB Function/1(pos_d) -> pos_d/1, Sum2/1
  switch2arm/1 -> Terminator/1
  LimitDesiredVelocity/1(v_d) -> Sum/1
  Selector3/1 -> Filter1/1, ReshapeDesiredVelocity/2(current_vel), Sum/2
  Sum2/1 -> PID Controller2/1, ReshapeDesiredVelocity/1(desired_vel)
  MISSION_MODE/1 -> Mission/3(MISSION_MODE)
  mission_point_num/1 -> Mission/2(mission_point_num)
  mission_point_list/1 -> Mission/1(mission_point_list)
  Gain1/1 -> LimitDesiredVelocity/1(desired_vel), Mission/4(manualRC), MATLAB Function/1(manualRC)
  Dead Zone1/1 -> Gain1/1
  deisred altitude updater/1(pz_d) -> Sum3/2
  Sum3/1 -> PID Controller3/1
  Selector1/1 -> Sum3/1, deisred altitude updater/2(pz)
  POS_ALT/1 -> PID Controller3/2
  PID Controller3/1 -> Add1/2
  PID Controller1/1 -> Add1/1
  POS_P/1 -> PID Controller2/2
  PID Controller2/1 -> Add/1
  PID Controller/1 -> Add/2
  Sum/1 -> PID Controller/1
  Selector/1 -> Mission/5(current_pos), MATLAB Function/2(current_pos), pos/1, Sum2/2
  Dead Zone/1 -> deisred altitude updater/1(S), Gain/1
  Mux/1 -> ad/1
  Add1/1 -> Mux/2
  Sum1/1 -> PID Controller1/1
  Selector2/1 -> Sum1/1
  Gain/1 -> Sum1/2
  Bias/1 -> Dead Zone/1
  throtte/1 -> Bias/1
  Add/1 -> Mux/1
  VEL_ALT/1 -> PID Controller1/2
  VEL_P/1 -> PID Controller/2
  v/1 -> Selector2/1, Selector3/1
  p/1 -> Selector1/1, Selector/1
  vhd/1 -> Dead Zone1/1

== matlab function FTC_UnknownV2/Subsystem2/MATLAB Function ==
  data: Reb input; eulerangle output
function eulerangle = fcn(Reb)
% 方位角计算
psi = atan2(Reb(2,1), Reb(1,1));
% 借助方位角快速计算出横滚俯仰角的余弦
costheta = Reb(1,1)/cos(psi);
cosphi = Reb(3,3)/costheta;
eulerangle = [psi; costheta; cosphi];

== matlab function FTC_UnknownV2/outerloop/Pos ==
  data: a_des_0 input single size=3; n3 input size=3; m input single size=1; fd output single size=1; g input single size=1; n3d output single size=[3,1]; ad output single size=3; SAT_AD input single size=1
function [fd, n3d, ad]  = fcn(a_des_0, n3, m, g, SAT_AD)
% 计算期望的主轴
    % a_des_g: 期望的电机产生总推力产生的加速度, 为了克服重力且重力方向是正方向所以推理克服重力应该是向上的,所以是-g 
    a_des_0_g = (a_des_0 - [single(0); single(0); g]);
    epsilon = max(  (sqrt(a_des_0_g(1)^2+a_des_0_g(2)^2)/abs(a_des_0_g(3)))/single(SAT_AD)  ,1);
    % 确保只压缩水平方向的加速度, 确保高度通道的加速的不会被饱和干扰, 做到真正的重力方向优先
    a_des_g = [1/epsilon 1/epsilon 1].*a_des_0_g';
    % 计算期望的主轴
    n3d = -(a_des_g')/norm(a_des_g);

    % 旧的方案
    % 计算饱和后的期望加速度
    ad = mysatsingle(a_des_0,single(SAT_AD)*g);
%     n3d = ([single(0); single(0); g]-ad)/norm([single(0); single(0); g]-ad);

% 计算期望的拉力
if n3d(3)==single(0)
    fd = single(0);
else
    % 旧方案
%     fd = m*(g-ad(3))/n3(3);
    % 新方案
    fd = m*(-a_des_g(3))/n3(3);

end

== matlab function FTC_UnknownV2/outerloop/Position2/deisred altitude updater ==
  data: S input; pz input; pz_d output
function pz_d = fcn(S, pz)
persistent pz_d_static
if isempty(pz_d_static)
    pz_d_static = single(0);
end

if abs(S) > 0.01
    pz_d_static = pz;
end
pz_d = pz_d_static;

== matlab function FTC_UnknownV2/outerloop/MATLAB Function1 ==
  data: u input; y output
function y = fcn(u)
y=diag([u,1,1,1]);

== matlab function FTC_UnknownV2/outerloop/d_z ==
  data: n3 input size=[3,1]; dvz input single size=1; T_ input single size=4; M input single size=[4,4]; m input single size=1; g input single size=1; dz output single size=1
function dz   = fcn(n3, dvz, T_, M, m, g)
dz  = m*(0.3*dvz-g)/n3(3)+M(1,:)*T_;

== matlab function FTC_UnknownV2/generate health matrix ==
  data: CH7 input; LOE input; Lambda output
function Lambda = fcn(CH7, LOE)
if LOE>0.3 %fault-free and 0.5 fault
    if LOE>0.8
        Lambda=diag([single(1),single(1),single(1),single(1)]);
    else
        Lambda=diag([single(0),single(1),single(1),single(1)]);
    end
else % one, two, and three rotors failure
    if CH7<1300
        Lambda=diag([single(0),single(0),single(1),single(1)]);
    else
        if CH7<1700 %1300<=CH7<1700
            Lambda=diag([single(0),single(1),single(0),single(1)]);
        else%CH7>=1700
            Lambda=diag([single(0),single(0),single(0),single(1)]);
        end
    end
end

== matlab function FTC_UnknownV2/outerloop/Position2/LimitDesiredVelocity ==
  data: desired_vel input; v_d output
function v_d = fcn(desired_vel)
v_d = mysatsingle(desired_vel,4);

== matlab function FTC_UnknownV2/innerloop/MATLAB Function3 ==
  data: n3 input; pqrd output; n3d input; Rbe input; ATT_P input
function pqrd = fcn(n3, n3d, Rbe,ATT_P)
% nc = cross(n3, n3d);
% ncb  = Rbe*nc;
e = n3 - n3d;
pqd = ATT_P*[-Rbe(1,2) Rbe(1,1);-Rbe(2,2) Rbe(2,1)]*[e(1);e(2)];
rd = 0;
pqrd = [pqd;rd];

== matlab function FTC_UnknownV2/outerloop/MATLAB Function4 ==
  data: u input; y output
function y = fcn(u)
y = [-u/5; 1]/norm([-u/5; 1]);

== matlab function FTC_UnknownV2/PX4 Time ==
  data: ts output
function ts  = fcn
% coder.cinclude('drivers/drv_hrt.h');
persistent count
if isempty(count)
    count = 0;
end

hrt = 0;
if coder.target('Rtw')
    hrt = coder.ceval('hrt_absolute_time');
else
    hrt = count;
end
ts = hrt;% us

count = count + 1;

== matlab function FTC_UnknownV2/quat2eul ==
  data: q input single; dcm output single
function dcm  = quat2eul(q)
% Conversion from Quaternion to Euler angles based on the PX4 Firmware
% v1.6.5 release.
% 
% Quaternion -> DCM -> Euler Angles
% INPUT:
%   q: Quaternion vector of the format: (a + bi + cj + dk)
% OUTPUT:
%   [phi,theta,psi]: Euler angles in radians.
% 
 if norm(q)~=0
    a = q(1);
    b = q(2);
    c = q(3);
    d = q(4);

    aSq = a*a;
    bSq = b*b;
    cSq = c*c;
    dSq = d*d;

    d_pi2 = pi/2;

    % quaternion_to_dcm
    dcm00 = aSq + bSq - cSq - dSq;
    dcm01 = 2*(b*c - a*d);
    dcm02 = 2*(a*c + b*d);
    dcm10 = 2*(b*c + a*d);
    dcm11 = aSq - bSq + cSq - dSq;
    dcm12 = 2*(c*d - a*b);
    dcm20 = 2*(b*d - a*c);
    dcm21 = 2*(a*b + c*d);
    dcm22 = aSq - bSq - cSq + dSq;
    dcm=[dcm00 dcm01 dcm02;
              dcm10 dcm11 dcm12;
              dcm20 dcm21  dcm22];
 else
     dcm = single(eye(3,3));
 end
    % dcm_to_euler

== matlab function FTC_UnknownV2/outerloop/Position2/ReshapeDesiredVelocity ==
  data: desired_vel input; v_d output; current_vel input
function v_d = fcn(desired_vel,current_vel)
v_d = genDesiredPos(current_vel,mysatsingle(desired_vel,0.5),[0;0],1,2);

== stateflow chart FTC_UnknownV2/outerloop/Position2/Mission ==
  state Init0
    entry: last_desired_pos = current_pos;
    current_desired_pos = current_pos;
    point_num_current = 1;
  state Manual
    during: p_des = current_pos + manualRC;
  state Mission_run
    entry: last_desired_pos = current_pos;
    current_desired_pos = mission_point_list(point_num_current,:)';
    during: p_des =genDesiredPos(current_pos, current_desired_pos,last_desired_pos,1,0.5);
  state Mission_stop
    during:p_des = current_desired_pos;
  (default) -> Init0
  Init0 -> Manual : [MISSION_MODE==1]
  Mission_stop -> Manual : [MISSION_MODE<=0.5]
      | {point_num_current = 1;}
  Mission_run -> Manual [order 1] : [MISSION_MODE<=0.5]
  Manual -> Mission_run : [MISSION_MODE>0.5]
  Mission_run -> Mission_stop [order 2] : [norm(current_pos-current_desired_pos)<1&point_num_current==mission_point_num]
  Mission_run -> Mission_run [order 3] : [norm(current_pos-current_desired_pos)<1]
      | {point_num_current = min(point_num_current+1,mission_point_num);}
  data: mission_point_list input; mission_point_num input; MISSION_MODE input; manualRC input; current_pos input; current_desired_pos local single; last_desired_pos local single; point_num_current local; p_des output

== matlab function FTC_UnknownV2/quat2eul1 ==
  data: q input single; dcm output single
function dcm  = quat2eul(q)
% Conversion from Quaternion to Euler angles based on the PX4 Firmware
% v1.6.5 release.
% 
% Quaternion -> DCM -> Euler Angles
% INPUT:
%   q: Quaternion vector of the format: (a + bi + cj + dk)
% OUTPUT:
%   [phi,theta,psi]: Euler angles in radians.
% 
 if norm(q)~=0
    a = q(1);
    b = q(2);
    c = q(3);
    d = q(4);

    aSq = a*a;
    bSq = b*b;
    cSq = c*c;
    dSq = d*d;

    d_pi2 = pi/2;

    % quaternion_to_dcm
    dcm00 = aSq + bSq - cSq - dSq;
    dcm01 = 2*(b*c - a*d);
    dcm02 = 2*(a*c + b*d);
    dcm10 = 2*(b*c + a*d);
    dcm11 = aSq - bSq + cSq - dSq;
    dcm12 = 2*(c*d - a*b);
    dcm20 = 2*(b*d - a*c);
    dcm21 = 2*(a*b + c*d);
    dcm22 = aSq - bSq - cSq + dSq;
    dcm=[dcm00 dcm01 dcm02;
              dcm10 dcm11 dcm12;
              dcm20 dcm21  dcm22];
 else
     dcm = single(eye(3,3));
 end
    % dcm_to_euler

== matlab function FTC_UnknownV2/innerloop/AttRate ==
  data: pqrd input; w input; dw input; T_ input; M input; RATE_P input; RATE_P_YAW input; J input; dpqr output size=3; taop output; taoq output; taor output; K_CP input
function [dpqr, taop, taoq, taor] = fcn(pqrd, w, dw, T_, M, RATE_P, RATE_P_YAW, J, K_CP)
pqd = pqrd(1:2);
rd    = pqrd(3);
%% 角速率控制器计算

k2 = RATE_P;
k2_scaled = k2*RATE_P_YAW;

% kr = 0.001;
% dp =  M(2,:)*T_ - J(1,1)*dw(1) - kr*abs(w(1))*w(1) + w(2)*w(3)*(J(2,2)-J(3,3));
% dq =  M(3,:)*T_ - J(2,2)*dw(2) - kr*abs(w(2))*w(2) + w(3)*w(1)*(J(3,3)-J(1,1));
% dr  =  M(4,:)*T_ - J(3,3)*dw(3) - kr*abs(w(3))*w(3) + w(1)*w(2)*(J(1,1)-J(2,2));
dp = M(2,:)*T_ -J(1,1)*dw(1) + w(2)*w(3)*(J(2,2)-J(3,3));
dq = M(3,:)*T_ -J(2,2)*dw(2) + w(3)*w(1)*(J(3,3)-J(1,1));
dr = M(4,:)*T_ -J(3,3)*dw(3);

% taop =            J(1,1)*k2*(pqd(1)-w(1)) + kr*abs(w(1))*w(1) - w(2)*w(3)*(J(2,2)-J(3,3))+dp;
% taoq =            J(2,2)*k2*(pqd(2)-w(2)) + kr*abs(w(2))*w(2) - w(3)*w(1)*(J(3,3)-J(1,1))+dq;
% taor  = mysatsingle(J(3,3)*k2_scaled*(rd-w(3)) + kr*abs(w(3))*w(3) - w(1)*w(2)*(J(1,1)-J(2,2))+dr,10.0);

% 叠加耦合项 -\omega\times J\omega
taop =           J(1,1)*k2*(pqd(1)-w(1)) - w(2)*w(3)*(J(2,2)-J(3,3)) + dp + K_CP*w(2)*w(3)*(J(2,2)-J(3,3));
taoq =           J(2,2)*k2*(pqd(2)-w(2)) - w(3)*w(1)*(J(3,3)-J(1,1)) + dq + K_CP*w(3)*w(1)*(J(3,3)-J(1,1));
taor  = mysatsingle(J(3,3)*k2_scaled*(rd-w(3))+ dr,1.0);

dpqr = [dp; dq; dr];

== matlab function FTC_UnknownV2/MATLAB Function4 ==
  data: x input; y2 output
function y2 = fcn(x)
p1 = 19.72;
p2 = -134.1;
p3 = 385.9;
y=p1*x.^2 + p2.*x + p3;
y2 = y.*x;

== matlab function FTC_UnknownV2/innerloop/fmincon ==
  data: fd input; taop input; taoq input; taor input; T output; T0 input; M input; val output; time output
function [T,val,time] = fcn(fd, taop, taoq, taor, T0, M)
%% 求解
w1= 1;
w2 =20;
w3= 20;
w4= 0.00;
myfun2 = @(x)(w1*(M(1,:)*x-fd)^2+w2*(M(2,:)*x-taop)^2+w3*(M(3,:)*x-taoq)^2+w4*(M(4,:)*x-taor)^2);

lb  = [0 0 0 0]';
ub  = [3 3 3 3]';

options = optimoptions(@fmincon,'Algorithm','sqp','MaxIterations',10);
% tic
[T,val] = fmincon(myfun2,T0,[],[],[],[],lb,ub,[],options);
% ff = toc;
time =0;

== matlab function FTC_UnknownV2/innerloop/quadprog ==
  data: fd input double; taop input double; taoq input double; taor input double; T output double; T0 input double; M input double; fval output double; iter output
function [T,fval, iter] = fcn(fd, taop, taoq, taor, T0, M)
%% 求解
vd = [fd; taop; taoq; taor];
W=diag([1 20 20 0.01]);
H = M'*W*M;
f = -(vd'*W*M)';
% Td = B*vd;
lb  = [0 0 0 0]';
ub  = [8.5 8.5 8.5 8.5]';
% if (max(B*vd)>3)||(min(B*vd)<0)
    options = optimoptions(@quadprog,'Algorithm','active-set','MaxIterations',10);

    [T,fval,~,output] = quadprog(H, f, [], [], [], [], lb, ub, T0, options);
     iter = output.iterations;
% else
%     T = B*vd;
%     fval = 0;
% end

== matlab function FTC_UnknownV2/innerloop/MATLAB Function1 ==
  data: u input; y output
function y = fcn(u)
y=diag([u,1,1,1]);

== matlab function FTC_UnknownV2/InputConditioning/MATLAB Function ==
  data: u input; y output
function y = fcn(u)

 if(u>1550)
    y=u;
 else
     if(u<1450)
     y=u;
     else
         y=single(1500);
     end
 end

== matlab function FTC_UnknownV2/InputConditioning/MATLAB Function1 ==
  data: u input; y output
function y = fcn(u)

 if(u>1550)
    y=u;
 else
     if(u<1450)
     y=u;
     else
         y=single(1500);
     end
 end

== matlab function FTC_UnknownV2/InputConditioning/MATLAB Function2 ==
  data: u input; y output
function y = fcn(u)

 if(u>1550)
    y=u;
 else
     if(u<1450)
     y=u;
     else
         y=single(1500);
     end
 end

== matlab function FTC_UnknownV2/MATLAB Function ==
  data: Lambda input; y output; fadePWM input
function y = fcn(Lambda, fadePWM)
s1 = Lambda(1,1) + Lambda(2,2) + Lambda(3,3) + Lambda(4,4);
if s1 ==1
    fadePWM(fadePWM==0)=170;
%     if(fadePWM(1)==0)
%         fadePWM(1) = 100;
%     end
%     if(fadePWM(1)==0)
%         fadePWM(1) = 100;
%     end
%     if(fadePWM(1)==0)
%         fadePWM(1) = 100;
%     end
%     if(fadePWM(4)==0)
%         fadePWM(4) = 100;
%     end
end
y = fadePWM+1000;

== matlab function FTC_UnknownV2/innerloop/Att ==
  data: e input; w input; eulerangle input; pqrd output; ATT_P input; ATT_P_SCALE input
function pqrd  = fcn(e, w, eulerangle, ATT_P, ATT_P_SCALE)
%% 角度控制1
% h1 = n3(1);
% h2 = n3(2);
% h3 = n3(3);
% h1d = n3d(1);
% h2d = n3d(2);
% h3d = n3d(3);
% we = Reb*w;
% k1 = single(5);
% epqd = [0 -1/h3; 1/h3 0]*[k1*(h1d-h1)+h2*we(3);k1*(h2d-h2)-h1*we(3)];
% 
% psid = single(0);
% rd = k1*0.3*(psid - psi);
% 
% Rbe = Reb';
% erd = (rd - Rbe(3,1)*epqd(1) - Rbe(3,2)*epqd(2))/Rbe(3,3);
% 
% pqd = Rbe((1:2),:)*[epqd; erd];%计算出机体系下的pqd
% pqd = mysat(pqd,2);
% pqrd = [pqd;rd];
%% 角度控制2
e1 = e(1);
e2 = e(2);
% e1  = n3(1) - n3d(1);
% e2  = n3(2) - n3d(2); 
beta = atan2(e2,e1);
psi = eulerangle(1);
costheta = eulerangle(2);
cosphi = eulerangle(3);
k1 = ATT_P;
pqd = [ -k1*sqrt(e1^2+e2^2)*sin(psi-beta);%costheta
             -k1*sqrt(e1^2+e2^2)*cos(psi-beta)];%cosphi
pqd = mysatsingle(pqd,3);
psid = 0;
% rd = -k1*0.3*(psi-psid);
rd = -k1*ATT_P_SCALE*(psi-psid);
% rd = 0;
pqrd = [pqd;rd];

== matlab function FTC_UnknownV2/innerloop/MATLAB Function2 ==
  data: pqd output; dpqr output; J input; Reb input; n3 input; n3d input; dn3d input; taop output; wf input; euler input; ATT_P_SCALE input; ATT_P input; dw input; T_ input; M input; K_CP input; RATE_P_YAW input; RATE_P input; taoq output; taor output
function [pqd,dpqr, taop, taoq, taor] = fcn(J, Reb, n3, n3d, dn3d, wf, euler, ATT_P_SCALE, ATT_P, dw, T_, M, K_CP, RATE_P_YAW, RATE_P)
A = Reb(1,1);
B = Reb(2,1);
C = Reb(1,2);
D = Reb(2,2);
E = Reb(3,1);
F = Reb(3,2);
n_3_x = Reb(1,3);
n_3_y = Reb(2,3);
n_3_z = Reb(3,3);
fx_1 = ([0 n_3_z;-n_3_z 0]*[A C;B D] + [-n_3_y;n_3_x]*[E F]);
K = ATT_P*[-B A;-D C];
G = -n_3_z*ATT_P*[1 0;0 1];
% For dotK
dReb = Reb*[0 -wf(3) wf(2);wf(3) 0 -wf(1);-wf(2) wf(1) 0];
dA = dReb(1,1);
dB = dReb(2,1);
dC = dReb(1,2);
dD = dReb(2,2);
dK = ATT_P*[-dB dA;-dD dC];
% For A_2
A_2 = [0 -wf(3)*(J(3,3)-J(2,2))/J(1,1);-wf(3)*(J(1,1)-J(3,3))/J(2,2) 0];

%% Controller
e = n3 - n3d;
% % Attitude Loop
%pqd = K*e(1:2);%期望主轴为常值的时候
pqd = K*e(1:2) + (K/ATT_P/(-n_3_z))*dn3d(1:2);%考虑期望的主轴为动态变化的时候
rd = -ATT_P*ATT_P_SCALE*(euler(1));
% % Rate Loop generating u_c
u_cpq = [J(1,1) 0;0 J(2,2)]*(-RATE_P*(wf(1:2)-pqd)-A_2*wf(1:2)-(fx_1'-dK-G*K)*e(1:2) + G*(wf(1:2)-pqd));%-(fx_1'-dK-G*K)*e(1:2) + G*(wf(1:2)-pqd)
u_cr  = J(3,3)*RATE_P*RATE_P_YAW*(rd-wf(3));

% Disturbance Estimate d
dp = M(2,:)*T_ -J(1,1)*dw(1) + wf(2)*wf(3)*(J(2,2)-J(3,3));
dq = M(3,:)*T_ -J(2,2)*dw(2) + wf(3)*wf(1)*(J(3,3)-J(1,1));
dr  = M(4,:)*T_ -J(3,3)*dw(3);
dpqr = [dp; dq; dr];

% u_0 = u_c + d
taop = u_cpq(1) + dp + K_CP*(wf(2) - pqd(2))*wf(3)*(J(2,2)-J(3,3));
taoq = u_cpq(2) + dq + K_CP*(wf(1) - pqd(1))*wf(3)*(J(3,3)-J(1,1));
taor = mysatsingle(u_cr + dr,1.0);

== matlab function FTC_UnknownV2/outerloop/Position2/MATLAB Function ==
  data: manualRC input; pos_d output; current_pos input; Ts input
function pos_d = fcn(manualRC, current_pos, Ts)
persistent desired_pos_static manualRC_last
if isempty(desired_pos_static)
    desired_pos_static = current_pos;
end
if isempty(manualRC_last)
    manualRC_last = single([0;0]);
end

if norm(manualRC)>0.01
    desired_pos_static = desired_pos_static + Ts*manualRC;
else
    if manualRC_last>0.01
        desired_pos_static = current_pos;
    end
end
manualRC_last = manualRC;
pos_d = desired_pos_static;
